simulink model "CSTR_01_AddMPCblk"  (R2025a)
settings: Solver=ode45  StartTime=0  StopTime=40  RelTol=1e-3  EnableMultiTasking=on
libraries: mpclib x1
settings Model: FPTRunName=Active  Creator=The MathWorks, Inc.  LastModifiedBy=amyyang
settings SolverCC: AlgebraicLoopSolver=TrustRegion  MaxZcPerStep=1.0
settings DataIOCC: InitialState=[311.267; 8.5695]  LimitDataPoints=on  SaveFormat=Array  ReturnWorkspaceOutputs=off  SignalLoggingName=logsOut
settings OptimizationCC: BooleanDataType=off  DefaultParameterBehavior=Inlined  InlineInvariantSignals=on  BufferReuse=off  ExpressionDepthLimit=2147483647.0  InitFltsAndDblsToZero=on  LifeSpan=inf
settings DebuggingCC: SaveWithParameterizedLinksMsg=none  UnderspecifiedInitializationDetection=Classic  MergeDetectMultiDrivingBlocksExec=none  CheckExecutionContextPreStartOutputMsg=on  SignalResolutionControl=TryResolveAllWithWarning  MultiTaskDSMMsg=warning  MultiTaskCondExecSysMsg=none  FcnCallInpInsideContextMsg=warning  UnconnectedInputMsg=warning  UnconnectedOutputMsg=warning  UnconnectedLineMsg=warning  StateNameClashWarn=warning  SFUnexpectedBacktrackingDiag=warning  SFNoUnconditionalDefaultTransitionDiag=warning  SFExecutionAtInitializationDiag=none  ArithmeticOperatorsInVariantConditions=warning
settings HardwareCC: ProdBitPerPointer=32.0  ProdBitPerSizeT=32.0  ProdBitPerPtrDiffT=32.0  ProdLargestAtomicFloat=None  ProdIntDivRoundTo=Undefined  ProdEndianess=Unspecified  ProdWordSize=32.0  ProdHWDeviceType=32-bit Generic  TargetUnknown=on
settings ModelReferenceCC: EnableRefExpFcnMdlSchedulingChecks=on  PropagateSignalLabelsOutOfModel=off
settings SFSimCC: SimUseLocalCustomCode=off  CustomCodeUndefinedFunction=UseInterfaceOnly
settings RTWCC: RTWUseLocalCustomCode=off  GPUComputeCapability=3.5  DLArmComputeVersion=19.05
settings CodeAppCC: StateflowObjectComments=on
settings GRTTargetCC: TargetFcnLib=ansi_tfl_tmw.mat  TargetLangStandard=C89/C90 (ANSI)  CombineOutputUpdateFcns=off  GRTInterface=on
settings ConfigComp: CovMetricSettings=dw  CovSaveCumulativeToWorkspaceVar=on  CovSaveSingleToWorkspaceVar=on  CovExternalEMLEnable=off

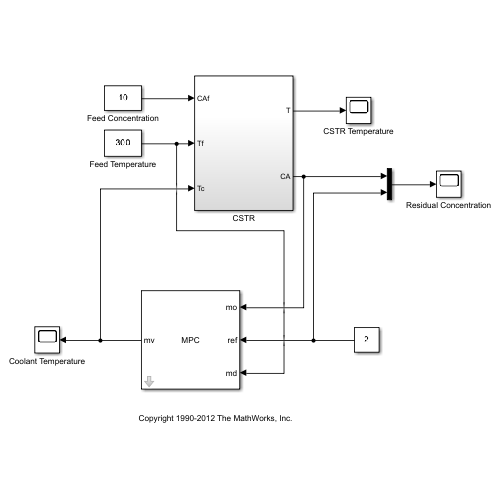
[thumbnail: Simulink's stored preview of the top-level diagram]
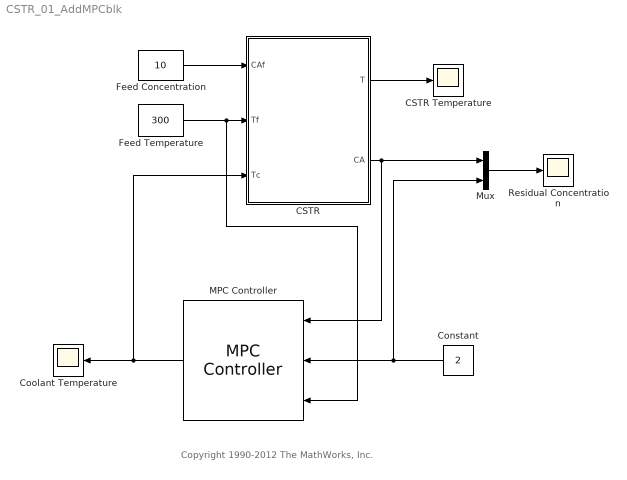
== system CSTR_01_AddMPCblk ==
  note: Copyright 1990-2012 The MathWorks, Inc.
  CSTR : Subsystem
  CSTR Temperature : Scope
      settings: ActiveDisplayYMinimum=280  ActiveDisplayYMaximum=320  DataLoggingVariableName=ScopeData2
  Constant : Constant  Value=2
  Coolant Temperature : Scope
      settings: ActiveDisplayYMinimum=280  ActiveDisplayYMaximum=320
  Feed Concentration : Constant  Value=10
  Feed Temperature : Constant  Value=300
  MPC Controller : mpclib/MPC Controller  SCDEnableBlockLinearizationSpecification=on  is_multiple=0  enable_value=0  return_u0=off  updateMPCinCallerWorkspace=on  md_inport=on  mv_inport=off  uref_inport=off  return_cost=off  return_mvseq=off  return_qpstatus=off  return_xseq=off  return_state=off  return_ovseq=off  state_inport=off  umin_inport=off  umax_inport=off  ymin_inport=off  ymax_inport=off  cc_inport=off  ywt_inport=off  uwt_inport=off  duwt_inport=off  rhoeps_inport=off  pm_inport=off  MaximumP=10  HorizonChoice=FixedHorizon  n_ts=0.1  n_p=10  n_mv=1  n_md=1  n_ud=1  n_mo=1  n_uo=0  BlockDataType=double  SampleTimeInherited=off  switch_inport=off
  Mux : Mux  Inputs=2
  Residual Concentration : Scope
      settings: ActiveDisplayYMinimum=8.3909492021760883  ActiveDisplayYMaximum=10.176457180415216
  wires:
  Feed Temperature/1 -> MPC Controller/3, CSTR/2(Tf)
  CSTR/1(T) -> CSTR Temperature/1
  Feed Concentration/1 -> CSTR/1(CAf)
  CSTR/2(CA) -> MPC Controller/1, Mux/1
  MPC Controller/1 -> CSTR/3(Tc), Coolant Temperature/1
  Constant/1 -> Mux/2, MPC Controller/2
  Mux/1 -> Residual Concentration/1

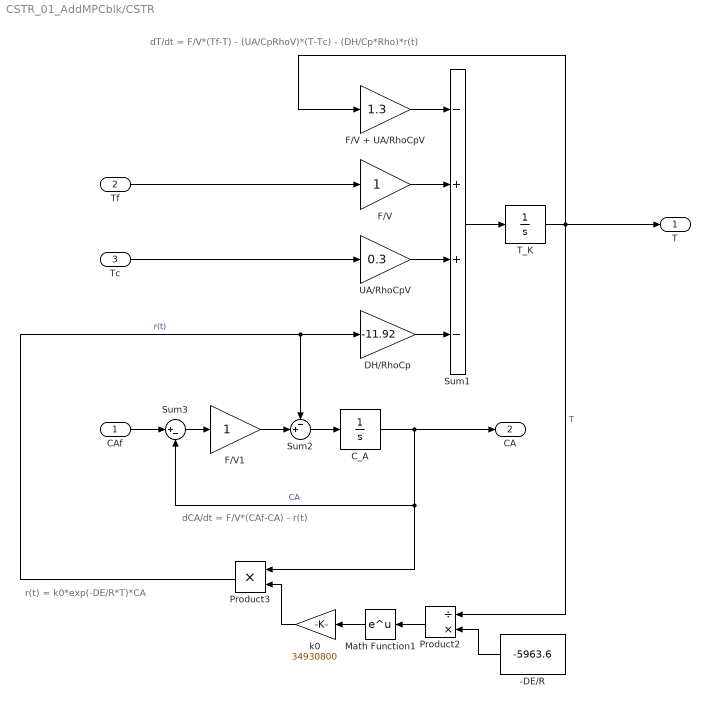
== system CSTR_01_AddMPCblk/CSTR ==
  note: dT/dt = F/V*(Tf-T) - (UA/CpRhoV)*(T-Tc) - (DH/Cp*Rho)*r(t)
  note: r(t) = k0*exp(-DE/R*T)*CA
  note: dCA/dt = F/V*(CAf-CA) - r(t)
  CAf : Inport
  Tf : Inport  Port=2
  Tc : Inport  Port=3
  -DE/R : Constant  Value=-5963.6  SampleTime=0
  C_A : Integrator  InitialCondition=8.5695  LimitOutput=on  LowerSaturationLimit=0
  DH/RhoCp : Gain  Gain=-11.92  SaturateOnIntegerOverflow=on  OutDataTypeStr=Inherit: Same as input  ParamDataTypeStr=Inherit: Same as input
  F/V : Gain  SaturateOnIntegerOverflow=on  OutDataTypeStr=Inherit: Same as input  ParamDataTypeStr=Inherit: Same as input
  F/V + UA/RhoCpV : Gain  Gain=1.3  SaturateOnIntegerOverflow=on  OutDataTypeStr=Inherit: Same as input  ParamDataTypeStr=Inherit: Same as input
  F/V1 : Gain  SaturateOnIntegerOverflow=on  OutDataTypeStr=Inherit: Same as input  ParamDataTypeStr=Inherit: Same as input
  Math Function1 : Math  SignedPower=on
  Product2 : Product  Inputs=/*  InputSameDT=on  RndMeth=Zero  SaturateOnIntegerOverflow=on  OutDataTypeStr=Inherit: Same as first input
  Product3 : Product  InputSameDT=on  RndMeth=Zero  SaturateOnIntegerOverflow=on  OutDataTypeStr=Inherit: Same as first input
  Sum1 : Sum  Inputs=-++-  InputSameDT=on  SaturateOnIntegerOverflow=on  OutDataTypeStr=Inherit: Same as first input
  Sum2 : Sum  Inputs=-+|
  Sum3 : Sum  Inputs=|+-
  T_K : Integrator  InitialCondition=311.267  LimitOutput=on  LowerSaturationLimit=0
  UA/RhoCpV : Gain  Gain=0.3  SaturateOnIntegerOverflow=on  OutDataTypeStr=Inherit: Same as input  ParamDataTypeStr=Inherit: Same as input
  k0 : Gain  Gain=34930800  SaturateOnIntegerOverflow=on  OutDataTypeStr=Inherit: Same as input  ParamDataTypeStr=Inherit: Same as input
  T : Outport
  CA : Outport  Port=2
  wires:
  UA/RhoCpV/1 -> Sum1/3
  Product2/1 -> Math Function1/1
  Product3/1 -> DH/RhoCp/1, Sum2/1  "r(t)"
  T_K/1 -> T/1, F/V + UA/RhoCpV/1, Product2/1  "T"
  Tf/1 -> F/V/1
  C_A/1 -> CA/1, Sum3/2, Product3/1  "CA"
  Sum3/1 -> F/V1/1
  F/V + UA/RhoCpV/1 -> Sum1/1
  F/V/1 -> Sum1/2
  F/V1/1 -> Sum2/2
  Sum1/1 -> T_K/1
  k0/1 -> Product3/2
  -DE/R/1 -> Product2/2
  Math Function1/1 -> k0/1
  DH/RhoCp/1 -> Sum1/4
  CAf/1 -> Sum3/1
  Sum2/1 -> C_A/1
  Tc/1 -> UA/RhoCpV/1
